simulink model "three_one_f"  (R2021b)
settings: Solver=VariableStepAuto  StartTime=0.0  StopTime=5.0  RelTol=1e-3
model workspace (MAT data in the model file):
  Kd = 0.0232044684912
  Ki = 40.135
  Kp = 1.27162060915
  b = 0.010556
  m = 0.00074944
libraries: simulink_extras x1
settings Model: Creator=sashaohayon  LastModifiedBy=parth
settings SolverCC: AlgebraicLoopSolver=TrustRegion
settings DebuggingCC: SFMachineParentedDataDiag=warning

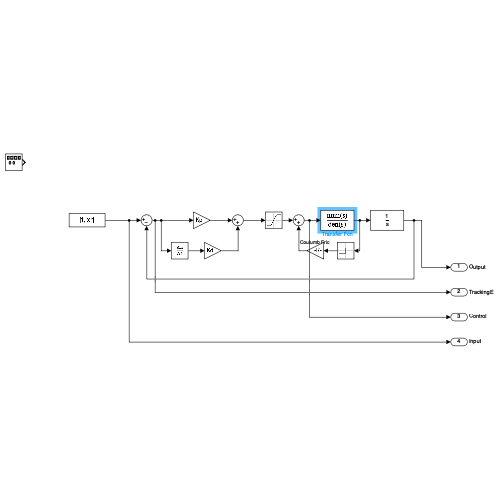
[thumbnail: Simulink's stored preview of the top-level diagram]
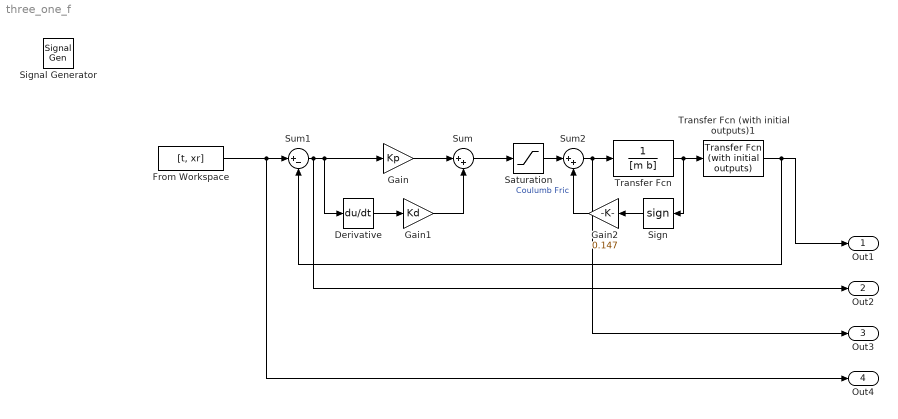
== system three_one_f ==
  Derivative : Derivative
  From Workspace : FromWorkspace  VariableName=[t, xr]
  Gain : Gain  Gain=Kp
  Gain1 : Gain  Gain=Kd
  Gain2 : Gain  Gain=0.147
  Saturation : Saturate  UpperLimit=8  LowerLimit=-8
  Sign : Signum
  Signal Generator : SignalGenerator  WaveForm=square  Frequency=0.5
  Sum : Sum  Inputs=|++
  Sum1 : Sum  Inputs=|+-
  Sum2 : Sum  Inputs=|++
  Transfer Fcn : TransferFcn  Denominator=[m b]
  Transfer Fcn (with initial outputs)1 : simulink_extras/Additional Linear/Transfer Fcn (with initial outputs)  N=[1]  D="[1  0]"  Y0=.5  U0=0
  Out1 : Outport  SignalName=Output
  Out2 : Outport  Port=2  SignalName=TrackingE
  Out3 : Outport  Port=3  SignalName=Control
  Out4 : Outport  Port=4  SignalName=Input
  wires:
  Gain/1 -> Sum/1
  Derivative/1 -> Gain1/1
  Gain1/1 -> Sum/2
  Transfer Fcn/1 -> Sign/1, Transfer Fcn (with initial outputs)1/1
  Transfer Fcn (with initial outputs)1/1 -> Out1/1, Sum1/2
  From Workspace/1 -> Out4/1, Sum1/1
  Sum1/1 -> Out2/1, Derivative/1, Gain/1
  Sum/1 -> Saturation/1
  Sign/1 -> Gain2/1
  Saturation/1 -> Sum2/1
  Sum2/1 -> Out3/1, Transfer Fcn/1
  Gain2/1 -> Sum2/2  "Coulumb Fric"
